simulink model "TwoLevelConverterIdealExample_HDL"  (R2023a)
settings: Solver=FixedStepAuto  StartTime=0.0  StopTime=0.1  RelTol=1e-3
PreLoadFcn:
  | ts = 1e-5; % local solver sample period
  | fsw = 1e3; % switching frequency
InitFcn:
  | load('stateSpaceParameters.mat');
undefined symbols (not defined in the file): DiscIntNeverNeededParam, ee_sli_rtmsupport, gcbh, stateSpaceParameters_1
libraries: fpga_utils_lib x5, hdlssclib x4, simulink x1, hdlsllib x1, eePwmGeneratorTwoLevel x1
settings Model: Creator=promero  LastModifiedBy=promero
settings OptimizationCC: BlockReduction=off  ConditionallyExecuteInputs=off  DefaultParameterBehavior=Inlined
settings DebuggingCC: AlgebraicLoopMsg=error
settings HardwareCC: ProdBitPerPointer=32  ProdBitPerSizeT=32  ProdBitPerPtrDiffT=32  ProdLargestAtomicFloat=None  ProdIntDivRoundTo=Undefined  ProdEndianess=Unspecified  ProdWordSize=32  ProdHWDeviceType=ASIC/FPGA->ASIC/FPGA  TargetBitPerPointer=64  TargetBitPerSizeT=64  TargetBitPerPtrDiffT=64  TargetLongLongMode=on  TargetIntDivRoundTo=Zero  TargetEndianess=LittleEndian  TargetWordSize=64  TargetHWDeviceType=Custom Processor->MATLAB Host Computer  ProdEqTarget=off

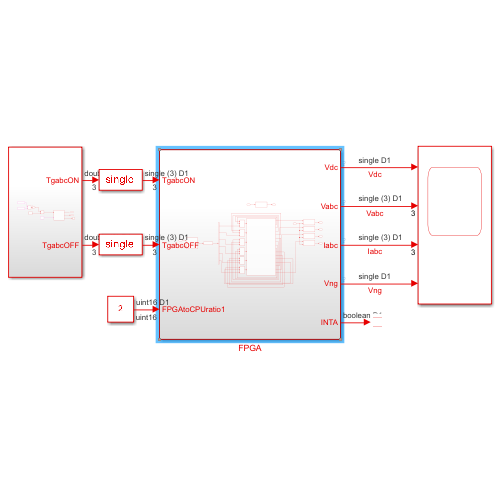
[thumbnail: Simulink's stored preview of the top-level diagram]
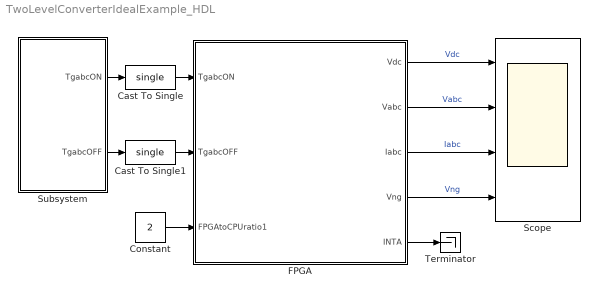
== system TwoLevelConverterIdealExample_HDL ==
  Cast To Single : DataTypeConversion  OutDataTypeStr=single  SaturateOnIntegerOverflow=off  RndMeth=Floor
  Cast To Single1 : DataTypeConversion  OutDataTypeStr=single  SaturateOnIntegerOverflow=off  RndMeth=Floor
  Constant : Constant  Value=2  OutDataTypeStr=uint16  SampleTime=-1
  FPGA : Subsystem
  Scope : Scope  NumInputPorts=4
  Subsystem : Subsystem
  Terminator : Terminator
  wires:
  FPGA/1(Vdc) -> Scope/1  "Vdc"
  FPGA/2(Vabc) -> Scope/2  "Vabc"
  FPGA/3(Iabc) -> Scope/3  "Iabc"
  FPGA/4(Vng) -> Scope/4  "Vng"
  Subsystem/1(TgabcON) -> Cast To Single/1
  Subsystem/2(TgabcOFF) -> Cast To Single1/1
  Cast To Single/1 -> FPGA/1(TgabcON)
  Cast To Single1/1 -> FPGA/2(TgabcOFF)
  FPGA/5(INTA) -> Terminator/1
  Constant/1 -> FPGA/3(FPGAtoCPUratio1)

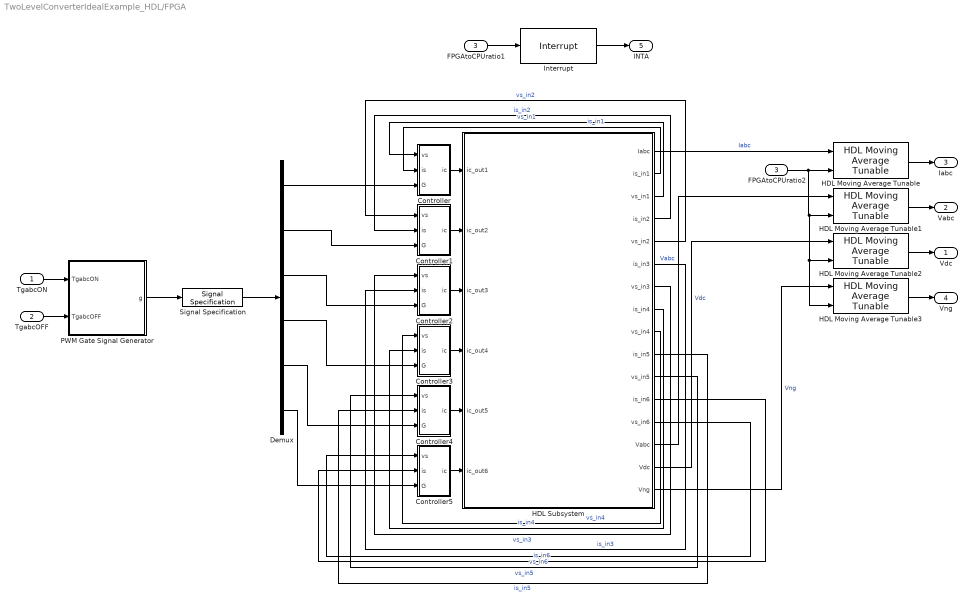
== system TwoLevelConverterIdealExample_HDL/FPGA ==
  TgabcON : Inport
  TgabcOFF : Inport  Port=2
  FPGAtoCPUratio1 : Inport  Port=3  OutDataTypeStr=uint16  LockScale=on
  Controller : Subsystem  mask{threshold=0.5, Gs=1e-6, s=1}
      mask prompts: Gs "Conductance (1/Ohm)"; s "Time scaling"
      mask DialogControl DescGroupVar Prompt: Description
      mask DialogControl Details Prompt: Switch Controller
  Controller1 : Subsystem  mask{threshold=0.5, Gs=1e-6, s=1}
      mask prompts: Gs "Conductance (1/Ohm)"; s "Time scaling"
      mask DialogControl DescGroupVar Prompt: Description
      mask DialogControl Details Prompt: Switch Controller
  Controller2 : Subsystem  mask{threshold=0.5, Gs=1e-6, s=1}
      mask prompts: Gs "Conductance (1/Ohm)"; s "Time scaling"
      mask DialogControl DescGroupVar Prompt: Description
      mask DialogControl Details Prompt: Switch Controller
  Controller3 : Subsystem  mask{threshold=0.5, Gs=1e-6, s=1}
      mask prompts: Gs "Conductance (1/Ohm)"; s "Time scaling"
      mask DialogControl DescGroupVar Prompt: Description
      mask DialogControl Details Prompt: Switch Controller
  Controller4 : Subsystem  mask{threshold=0.5, Gs=1e-6, s=1}
      mask prompts: Gs "Conductance (1/Ohm)"; s "Time scaling"
      mask DialogControl DescGroupVar Prompt: Description
      mask DialogControl Details Prompt: Switch Controller
  Controller5 : Subsystem  mask{threshold=0.5, Gs=1e-6, s=1}
      mask prompts: Gs "Conductance (1/Ohm)"; s "Time scaling"
      mask DialogControl DescGroupVar Prompt: Description
      mask DialogControl Details Prompt: Switch Controller
  Demux : Demux  Outputs=6
  FPGAtoCPUratio2 : InportShadow  Port=3  OutDataTypeStr=uint16
      settings: LockScale=on
  HDL Moving Average Tunable{,1..3} (4 alike) : fpga_utils_lib/HDL Moving Average Tunable  SystemSampleTime=-1  VariantActivationTime=update diagram  Latency=0  AutoFrameSizeCalculation=off
  HDL Subsystem : Subsystem  VariantControl=HDLSubsys
  Interrupt : fpga_utils_lib/Interrupt  SystemSampleTime=-1  VariantActivationTime=update diagram  Latency=0  AutoFrameSizeCalculation=off
  PWM Gate Signal Generator : Subsystem  Variant=on  VariantControlMode=label  VariantControl=Choice  LabelModeActiveChoice=hdlVar
  Signal Specification : SignalSpecification  OutDataTypeStr=boolean
      settings: LockScale=on
  Vdc : Outport
  Vabc : Outport  Port=2
  Iabc : Outport  Port=3
  Vng : Outport  Port=4
  INTA : Outport  Port=5
  wires:
  HDL Subsystem/3(vs_in1) -> Controller/1(vs)  "vs_in1"
  HDL Subsystem/7(vs_in3) -> Controller2/1(vs)  "vs_in3"
  Controller4/1(ic) -> HDL Subsystem/5(ic_out5)
  HDL Subsystem/5(vs_in2) -> Controller1/1(vs)  "vs_in2"
  Controller2/1(ic) -> HDL Subsystem/3(ic_out3)
  Controller/1(ic) -> HDL Subsystem/1(ic_out1)
  HDL Subsystem/2(is_in1) -> Controller/2(is)  "is_in1"
  HDL Subsystem/9(vs_in4) -> Controller3/1(vs)  "vs_in4"
  HDL Subsystem/12(is_in6) -> Controller5/2(is)  "is_in6"
  Controller5/1(ic) -> HDL Subsystem/6(ic_out6)
  Controller3/1(ic) -> HDL Subsystem/4(ic_out4)
  HDL Subsystem/4(is_in2) -> Controller1/2(is)  "is_in2"
  Controller1/1(ic) -> HDL Subsystem/2(ic_out2)
  Demux/1 -> Controller/3(G)
  HDL Subsystem/6(is_in3) -> Controller2/2(is)  "is_in3"
  HDL Subsystem/8(is_in4) -> Controller3/2(is)  "is_in4"
  HDL Subsystem/11(vs_in5) -> Controller4/1(vs)  "vs_in5"
  Demux/2 -> Controller1/3(G)
  HDL Subsystem/10(is_in5) -> Controller4/2(is)  "is_in5"
  Demux/3 -> Controller2/3(G)
  HDL Subsystem/13(vs_in6) -> Controller5/1(vs)  "vs_in6"
  Demux/6 -> Controller5/3(G)
  Demux/4 -> Controller3/3(G)
  Demux/5 -> Controller4/3(G)
  TgabcON/1 -> PWM Gate Signal Generator/1(TgabcON)
  TgabcOFF/1 -> PWM Gate Signal Generator/2(TgabcOFF)
  PWM Gate Signal Generator/1(g) -> Signal Specification/1
  Signal Specification/1 -> Demux/1
  Interrupt/1 -> INTA/1
  FPGAtoCPUratio1/1 -> Interrupt/1
  HDL Subsystem/1(Iabc) -> HDL Moving Average Tunable/1  "Iabc"
  FPGAtoCPUratio2/1 -> HDL Moving Average Tunable3/2, HDL Moving Average Tunable2/2, HDL Moving Average Tunable1/2, HDL Moving Average Tunable/2
  HDL Moving Average Tunable/1 -> Iabc/1
  HDL Subsystem/14(Vabc) -> HDL Moving Average Tunable1/1  "Vabc"
  HDL Subsystem/15(Vdc) -> HDL Moving Average Tunable2/1  "Vdc"
  HDL Subsystem/16(Vng) -> HDL Moving Average Tunable3/1  "Vng"
  HDL Moving Average Tunable1/1 -> Vabc/1
  HDL Moving Average Tunable2/1 -> Vdc/1
  HDL Moving Average Tunable3/1 -> Vng/1

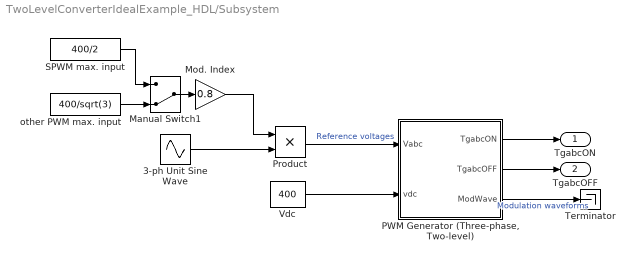
== system TwoLevelConverterIdealExample_HDL/Subsystem ==
  3-ph Unit Sine Wave : Sin  Frequency=2*pi*60  Phase="[0  -2*pi/3  2*pi/3] + pi/2"  SampleTime=ts
  Manual Switch1 : ManualSwitch  CurrentSetting=0
  Mod. Index : Gain  Gain=0.8
  "PWM Generator (Three-phase, Two-level)" : Subsystem  AncestorBlock=|  LoadFcn=ee_sli_rtmsupport( 'loadfcn', gcbh );  mask(PWM Generator (three-phase, two-level)){PWMMode=Continuous PWM (CPWM), CPWMMode=SVM: space vector modulation, DPWMMode=120 DPWM: positive dc component, SamplingMode=Natural, fsw=fsw, Ts=ts}
      | eePwmGeneratorTwoLevel/PWM Generator
      | (Three-phase, Two-level)
      mask prompts: PWMMode "physmod:ee:library:comments:control:eePwmGeneratorTwoLevel:PWMMode_MP"; CPWMMode "physmod:ee:library:comments:control:eePwmGeneratorTwoLevel:ContinuousPWM_MP"; DPWMMode "physmod:ee:library:comments:control:eePwmGeneratorTwoLevel:DiscontinuousPWM_MP"; SamplingMode "physmod:ee:library:comments:control:eePwmGeneratorTwoLevel:SamplingMode_MP"; fsw "physmod:ee:library:comments:control:eePwmGeneratorTwoLevel:SwitchingFrequencyHz_MP"; Ts "physmod:ee:library:comments:control:eePwmGeneratorTwoLevel:SampleTimes_MP"
      mask help: physmod:ee:library:comments:control:eePwmGeneratorTwoLevel:PWMGeneratorthreephaseTwolevel_MD
      mask init:
      | Tsw = 1/fsw;
      | 
      | if fsw <= 0
      |     error(message('physmod:simscape:compiler:patterns:checks:GreaterThanZero',getString(message('physmod:ee:library:comments:control:eePwmGeneratorTwoLevel:SwitchingFrequencyHz_MP'))));
      | end
      | 
      | if Ts <= 0
      |     error(message('physmod:simscape:compiler:patterns:checks:GreaterThanZero',getString(message('physmod:ee:library:comments:control:eePwmGeneratorTwoLevel:SampleTimes_MP'))));
      | end
      | 
      | if Ts > 1/(10*fsw)
      |     error(message('physmod:simscape:compiler:patterns:checks:LessThanOrEqual',getString(message('physmod:ee:library:comments:control:eePwmGeneratorTwoLevel:SampleTimes_MP')),getString(message('physmod:ee:library:comments:control:eePwmGeneratorTwoLevel:inverseOf10TimesSwitchingFrequency_MP'))));
      | end
      | 
      | switch SamplingMode
      |     case 'Natural'
      |         RateTransitionOnInput = -1;
      |         GateGeneratorX0 = 0;
      |     case 'Asymmetric'
      |         RateTransitionOnInput = 0.5*Tsw;
      |         GateGeneratorX0 = 0.5/fsw;
      |     case 'Symmetric'
      |         RateTransitionOnInput = Tsw;
      |         GateGeneratorX0 = 0;
      | end
      | 
      | 
      | switch PWMMode
      |     case 'Continuous PWM (CPWM)'
      |         switch CPWMMode
      |             case 'SPWM: sinusoidal PWM'
      |                 PWM = 1;
      |             case 'SVM: space vector modulation'
      |                 PWM = 2;
      |         end
      |     case 'Discontinuous PWM (DPWM)'
      |         switch DPWMMode
      |             case '60 DPWM: 60 degree discontinuous PWM'
      |                 PWM = 3;
      |             case '60 DPWM (+30 degree shift): +30 degree shift from 60 DPWM'
      |                 PWM = 4;
      |             case '60 DPWM (-30 degree shift): -30 degree shift from 60 DPWM'
      |                 PWM = 5;
      |             case '30 DPWM: 30 degree discontinuous PWM'
      |                 PWM = 6;
      |             case '120 DPWM: positive dc component'
      |                 PWM = 7;
      |             case '120 DPWM: negative dc component'
      |                 PWM = 8;
      |         end
      | end
      settings: CopyFcn=ee_sli_rtmsupport( 'copyfcn', gcbh );  DeleteFcn=ee_sli_rtmsupport( 'deletefcn', gcbh );  ModelCloseFcn=ee_sli_rtmsupport( 'modelclosefcn', gcbh );  PreSaveFcn=%pe_sli_rtmsupport( 'presavefcn', gcbh );  PostSaveFcn=ee_sli_rtmsupport( 'postsavefcn', gcbh );  PreCopyFcn=ee_sli_rtmsupport( 'precopyfcn', gcbh );  OpenFcn=ee_sli_rtmsupport( 'openfcn', gcbh );  CloseFcn=ee_sli_rtmsupport( 'closefcn', gcbh );  PreDeleteFcn=ee_sli_rtmsupport( 'predeletefcn', gcbh );
      settings: LibrarySourceBlock=|
      | eePwmGeneratorTwoLevel/PWM Generator
      | (Three-phase, Two-level)
      mask Help: web(nesl_help(gcbh))
      mask TypeOptions PWMMode: physmod:ee:library:comments:control:eePwmGeneratorTwoLevel:ContinuousPWMCPWM_PV | physmod:ee:library:comments:control:eePwmGeneratorTwoLevel:DiscontinuousPWMDPWM_PV
      mask Callback PWMMode:
      | switch get_param(gcb,'PWMMode')
      |     case 'Continuous PWM (CPWM)'
      |         set_param(gcb,'MaskVisibilities',{'on';'on';'off';'on';'on';'on'})
      |     case 'Discontinuous PWM (DPWM)'
      |         set_param(gcb,'MaskVisibilities',{'on';'off';'on';'on';'on';'on'})
      | end
      mask TypeOptions CPWMMode: physmod:ee:library:comments:control:eePwmGeneratorTwoLevel:SPWMSinusoidalPWM_PV | physmod:ee:library:comments:control:eePwmGeneratorTwoLevel:SVMSpaceVectorModulation_PV
      mask TypeOptions DPWMMode: physmod:ee:library:comments:control:eePwmGeneratorTwoLevel:x60DPWM60DegreeDiscontinuousPWM_PV | physmod:ee:library:comments:control:eePwmGeneratorTwoLevel:x60DPWM30DegreeShift30DegreeShiftFrom60DPWM_PV | physmod:ee:library:comments:control:eePwmGeneratorTwoLevel:x60DPWM0x2D30DegreeShift0x2D30DegreeShiftFrom60DPWM_PV | physmod:ee:library:comments:control:eePwmGeneratorTwoLevel:x30DPWM30DegreeDiscontinuousPWM_PV | physmod:ee:library:comments:control:eePwmGeneratorTwoLevel:x120DPWMPositiveDcComponent_PV | physmod:ee:library:comments:control:eePwmGeneratorTwoLevel:x120DPWMNegativeDcComponent_PV
      mask TypeOptions SamplingMode: physmod:ee:library:comments:control:eePwmGeneratorTwoLevel:Natural_PV | physmod:ee:library:comments:control:eePwmGeneratorTwoLevel:Asymmetric_PV | physmod:ee:library:comments:control:eePwmGeneratorTwoLevel:Symmetric_PV
      mask DialogControl ParameterGroupVar Prompt: physmod:ee:library:comments:control:eePwmGeneratorTwoLevel:tab_Parameters
      mask DialogControl PWMMode Prompt: PWM mode
      mask DialogControl CPWMMode Prompt: Continuous PWM
      mask DialogControl DPWMMode Prompt: Discontinuous PWM
      mask DialogControl SamplingMode Prompt: Sampling mode
      mask DialogControl fsw Prompt: Switching frequency (Hz)
      mask DialogControl Ts Prompt: Sample time (s)
  Product : Product
  SPWM max. input : Constant  Value=400/2
  Terminator : Terminator
  Vdc : Constant  Value=400
  other PWM max. input : Constant  Value=400/sqrt(3)
  TgabcON : Outport
  TgabcOFF : Outport  Port=2
  wires:
  Product/1 -> "PWM Generator (Three-phase, Two-level)"/1(Vabc)  "Reference voltages"
  Vdc/1 -> "PWM Generator (Three-phase, Two-level)"/2(vdc)
  other PWM max. input/1 -> Manual Switch1/2
  SPWM max. input/1 -> Manual Switch1/1
  Manual Switch1/1 -> Mod. Index/1
  "PWM Generator (Three-phase, Two-level)"/3(ModWave) -> Terminator/1  "Modulation waveforms"
  Mod. Index/1 -> Product/1
  3-ph Unit Sine Wave/1 -> Product/2
  "PWM Generator (Three-phase, Two-level)"/2(TgabcOFF) -> TgabcOFF/1
  "PWM Generator (Three-phase, Two-level)"/1(TgabcON) -> TgabcON/1

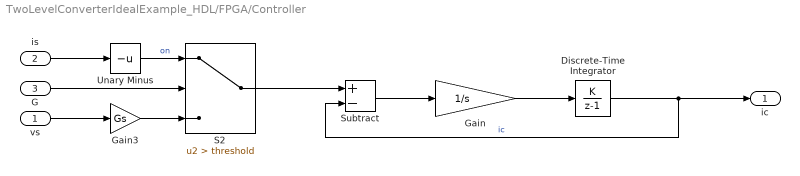
== system TwoLevelConverterIdealExample_HDL/FPGA/Controller ==
  vs : Inport
  is : Inport  Port=2
  G : Inport  Port=3
  Discrete-Time Integrator : DiscreteIntegrator  IntegratorMethod=Accumulation: Forward Euler  SampleTime=-1  ICPrevOutput=DiscIntNeverNeededParam  ICPrevScaledInput=DiscIntNeverNeededParam
  Gain : Gain  Gain=1/s
  Gain3 : Gain  Gain=Gs
  S2 : Switch  Criteria=u2 > Threshold  Threshold=threshold  SaturateOnIntegerOverflow=off  InputSameDT=off
  Subtract : Sum  Inputs=+-
  Unary Minus : UnaryMinus
  ic : Outport
  wires:
  G/1 -> S2/2
  is/1 -> Unary Minus/1
  Discrete-Time Integrator/1 -> Subtract/2, ic/1  "ic"
  Subtract/1 -> Gain/1
  Gain/1 -> Discrete-Time Integrator/1
  vs/1 -> Gain3/1
  S2/1 -> Subtract/1
  Gain3/1 -> S2/3
  Unary Minus/1 -> S2/1  "on"

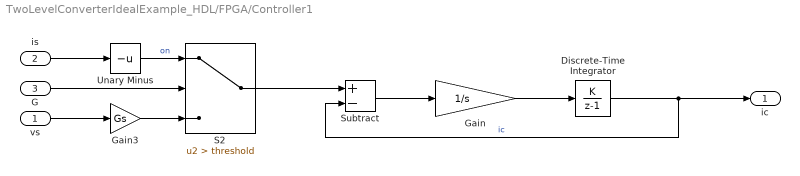
== system TwoLevelConverterIdealExample_HDL/FPGA/Controller1 ==
  vs : Inport
  is : Inport  Port=2
  G : Inport  Port=3
  Discrete-Time Integrator : DiscreteIntegrator  IntegratorMethod=Accumulation: Forward Euler  SampleTime=-1  ICPrevOutput=DiscIntNeverNeededParam  ICPrevScaledInput=DiscIntNeverNeededParam
  Gain : Gain  Gain=1/s
  Gain3 : Gain  Gain=Gs
  S2 : Switch  Criteria=u2 > Threshold  Threshold=threshold  SaturateOnIntegerOverflow=off  InputSameDT=off
  Subtract : Sum  Inputs=+-
  Unary Minus : UnaryMinus
  ic : Outport
  wires:
  Unary Minus/1 -> S2/1  "on"
  Gain3/1 -> S2/3
  S2/1 -> Subtract/1
  vs/1 -> Gain3/1
  Gain/1 -> Discrete-Time Integrator/1
  Subtract/1 -> Gain/1
  Discrete-Time Integrator/1 -> ic/1, Subtract/2  "ic"
  is/1 -> Unary Minus/1
  G/1 -> S2/2

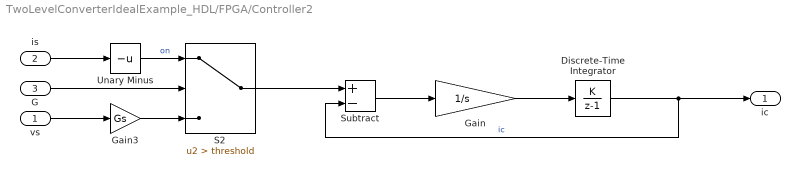
== system TwoLevelConverterIdealExample_HDL/FPGA/Controller2 ==
  vs : Inport
  is : Inport  Port=2
  G : Inport  Port=3
  Discrete-Time Integrator : DiscreteIntegrator  IntegratorMethod=Accumulation: Forward Euler  SampleTime=-1  ICPrevOutput=DiscIntNeverNeededParam  ICPrevScaledInput=DiscIntNeverNeededParam
  Gain : Gain  Gain=1/s
  Gain3 : Gain  Gain=Gs
  S2 : Switch  Criteria=u2 > Threshold  Threshold=threshold  SaturateOnIntegerOverflow=off  InputSameDT=off
  Subtract : Sum  Inputs=+-
  Unary Minus : UnaryMinus
  ic : Outport
  wires:
  Unary Minus/1 -> S2/1  "on"
  Gain3/1 -> S2/3
  S2/1 -> Subtract/1
  vs/1 -> Gain3/1
  Gain/1 -> Discrete-Time Integrator/1
  Subtract/1 -> Gain/1
  Discrete-Time Integrator/1 -> ic/1, Subtract/2  "ic"
  is/1 -> Unary Minus/1
  G/1 -> S2/2

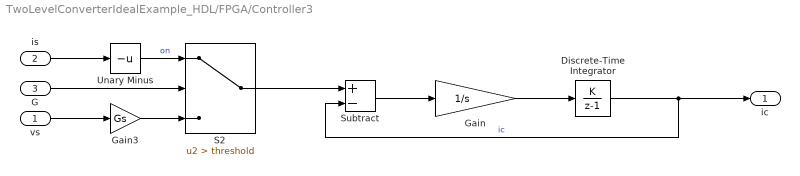
== system TwoLevelConverterIdealExample_HDL/FPGA/Controller3 ==
  vs : Inport
  is : Inport  Port=2
  G : Inport  Port=3
  Discrete-Time Integrator : DiscreteIntegrator  IntegratorMethod=Accumulation: Forward Euler  SampleTime=-1  ICPrevOutput=DiscIntNeverNeededParam  ICPrevScaledInput=DiscIntNeverNeededParam
  Gain : Gain  Gain=1/s
  Gain3 : Gain  Gain=Gs
  S2 : Switch  Criteria=u2 > Threshold  Threshold=threshold  SaturateOnIntegerOverflow=off  InputSameDT=off
  Subtract : Sum  Inputs=+-
  Unary Minus : UnaryMinus
  ic : Outport
  wires:
  G/1 -> S2/2
  is/1 -> Unary Minus/1
  Discrete-Time Integrator/1 -> Subtract/2, ic/1  "ic"
  Subtract/1 -> Gain/1
  Gain/1 -> Discrete-Time Integrator/1
  vs/1 -> Gain3/1
  S2/1 -> Subtract/1
  Gain3/1 -> S2/3
  Unary Minus/1 -> S2/1  "on"

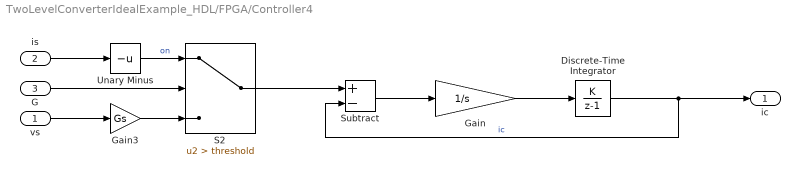
== system TwoLevelConverterIdealExample_HDL/FPGA/Controller4 ==
  vs : Inport
  is : Inport  Port=2
  G : Inport  Port=3
  Discrete-Time Integrator : DiscreteIntegrator  IntegratorMethod=Accumulation: Forward Euler  SampleTime=-1  ICPrevOutput=DiscIntNeverNeededParam  ICPrevScaledInput=DiscIntNeverNeededParam
  Gain : Gain  Gain=1/s
  Gain3 : Gain  Gain=Gs
  S2 : Switch  Criteria=u2 > Threshold  Threshold=threshold  SaturateOnIntegerOverflow=off  InputSameDT=off
  Subtract : Sum  Inputs=+-
  Unary Minus : UnaryMinus
  ic : Outport
  wires:
  G/1 -> S2/2
  is/1 -> Unary Minus/1
  Discrete-Time Integrator/1 -> Subtract/2, ic/1  "ic"
  Subtract/1 -> Gain/1
  Gain/1 -> Discrete-Time Integrator/1
  vs/1 -> Gain3/1
  S2/1 -> Subtract/1
  Gain3/1 -> S2/3
  Unary Minus/1 -> S2/1  "on"

== system TwoLevelConverterIdealExample_HDL/FPGA/Controller5 ==
  vs : Inport
  is : Inport  Port=2
  G : Inport  Port=3
  Discrete-Time Integrator : DiscreteIntegrator  IntegratorMethod=Accumulation: Forward Euler  SampleTime=-1  ICPrevOutput=DiscIntNeverNeededParam  ICPrevScaledInput=DiscIntNeverNeededParam
  Gain : Gain  Gain=1/s
  Gain3 : Gain  Gain=Gs
  S2 : Switch  Criteria=u2 > Threshold  Threshold=threshold  SaturateOnIntegerOverflow=off  InputSameDT=off
  Subtract : Sum  Inputs=+-
  Unary Minus : UnaryMinus
  ic : Outport
  wires:
  Unary Minus/1 -> S2/1  "on"
  Gain3/1 -> S2/3
  S2/1 -> Subtract/1
  vs/1 -> Gain3/1
  Gain/1 -> Discrete-Time Integrator/1
  Subtract/1 -> Gain/1
  Discrete-Time Integrator/1 -> ic/1, Subtract/2  "ic"
  is/1 -> Unary Minus/1
  G/1 -> S2/2

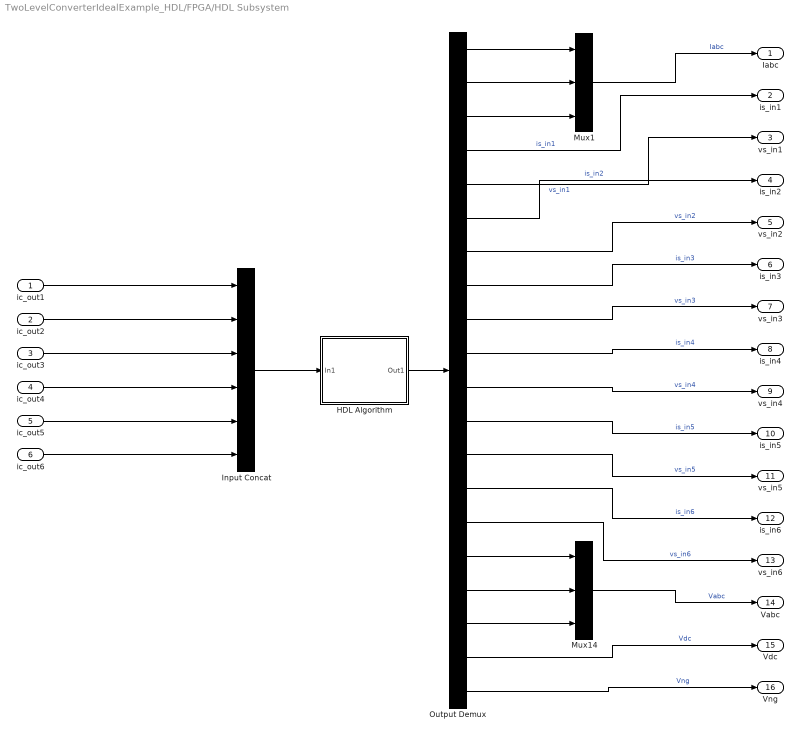
== system TwoLevelConverterIdealExample_HDL/FPGA/HDL Subsystem ==
  ic_out1 : Inport
  ic_out2 : Inport  Port=2
  ic_out3 : Inport  Port=3
  ic_out4 : Inport  Port=4
  ic_out5 : Inport  Port=5
  ic_out6 : Inport  Port=6
  HDL Algorithm : Subsystem  Variant=on  VariantControlMode=label  VariantControl=Choice  LabelModeActiveChoice=StateSpaceBlock
  Input Concat : Concatenate  NumInputs=6
  Mux1 : Mux  Inputs=3
  Mux14 : Mux  Inputs=3
  Output Demux : Demux  Outputs=20
  Iabc : Outport
  is_in1 : Outport  Port=2
  vs_in1 : Outport  Port=3
  is_in2 : Outport  Port=4
  vs_in2 : Outport  Port=5
  is_in3 : Outport  Port=6
  vs_in3 : Outport  Port=7
  is_in4 : Outport  Port=8
  vs_in4 : Outport  Port=9
  is_in5 : Outport  Port=10
  vs_in5 : Outport  Port=11
  is_in6 : Outport  Port=12
  vs_in6 : Outport  Port=13
  Vabc : Outport  Port=14
  Vdc : Outport  Port=15
  Vng : Outport  Port=16
  wires:
  Output Demux/7 -> vs_in2/1  "vs_in2"
  ic_out1/1 -> Input Concat/1
  Output Demux/18 -> Mux14/3
  Output Demux/17 -> Mux14/2
  Output Demux/16 -> Mux14/1
  Output Demux/13 -> vs_in5/1  "vs_in5"
  Output Demux/5 -> vs_in1/1  "vs_in1"
  Output Demux/2 -> Mux1/2
  Output Demux/19 -> Vdc/1  "Vdc"
  Output Demux/3 -> Mux1/3
  Output Demux/1 -> Mux1/1
  Output Demux/8 -> is_in3/1  "is_in3"
  Output Demux/10 -> is_in4/1  "is_in4"
  Mux1/1 -> Iabc/1  "Iabc"
  Output Demux/9 -> vs_in3/1  "vs_in3"
  Output Demux/15 -> vs_in6/1  "vs_in6"
  Output Demux/6 -> is_in2/1  "is_in2"
  Output Demux/4 -> is_in1/1  "is_in1"
  Output Demux/20 -> Vng/1  "Vng"
  ic_out3/1 -> Input Concat/3
  ic_out4/1 -> Input Concat/4
  ic_out5/1 -> Input Concat/5
  ic_out2/1 -> Input Concat/2
  Output Demux/11 -> vs_in4/1  "vs_in4"
  Output Demux/14 -> is_in6/1  "is_in6"
  Output Demux/12 -> is_in5/1  "is_in5"
  Mux14/1 -> Vabc/1  "Vabc"
  ic_out6/1 -> Input Concat/6
  Input Concat/1 -> HDL Algorithm/1(In1)
  HDL Algorithm/1(Out1) -> Output Demux/1

== system TwoLevelConverterIdealExample_HDL/FPGA/PWM Gate Signal Generator ==
  TgabcON : Inport
  TgabcOFF : Inport  Port=2
  HDL counter : Subsystem  VariantControl=hdlVar
      settings: LibrarySourceBlock=|
      | ee_sl_lib/Pulse Width
      | Modulation/PWM Gate Signal Generator
      | (Three-phase, Two-level)
  Off-the-shelf block : eePwmGeneratorTwoLevel/PWM Gate Signal Generator (Three-phase, Two-level)  VariantControl=defVar  fsw=fsw  Ts=ts
      settings: SamplingMode=Natural
      settings: LibrarySourceBlock=|
      | ee_sl_lib/Pulse Width
      | Modulation/PWM Gate Signal Generator
      | (Three-phase, Two-level)
  g : Outport

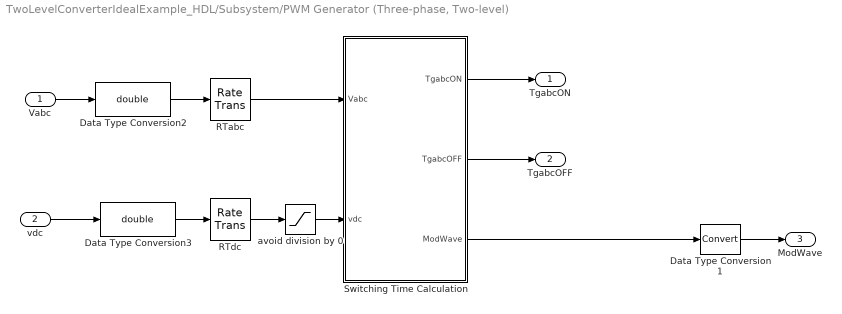
== system TwoLevelConverterIdealExample_HDL/Subsystem/PWM Generator (Three-phase, Two-level) ==
  Vabc : Inport
  vdc : Inport  Port=2
  Data Type Conversion1 : DataTypeConversion  SaturateOnIntegerOverflow=off  RndMeth=Floor
  Data Type Conversion2 : DataTypeConversion  OutDataTypeStr=double  SaturateOnIntegerOverflow=off  RndMeth=Floor
  Data Type Conversion3 : DataTypeConversion  OutDataTypeStr=double  SaturateOnIntegerOverflow=off  RndMeth=Floor
  RTabc : RateTransition  OutPortSampleTime=RateTransitionOnInput
  RTdc : RateTransition  OutPortSampleTime=RateTransitionOnInput
  Switching Time Calculation : MATLAB Function  TreatAsAtomicUnit=on
  avoid division by 0 : Saturate  UpperLimit=inf  LowerLimit=eps
  TgabcON : Outport
  TgabcOFF : Outport  Port=2
  ModWave : Outport  Port=3  VectorParamsAs1DForOutWhenUnconnected=off
  wires:
  Data Type Conversion3/1 -> RTdc/1
  Data Type Conversion2/1 -> RTabc/1
  vdc/1 -> Data Type Conversion3/1
  Vabc/1 -> Data Type Conversion2/1
  Switching Time Calculation/1(TgabcON) -> TgabcON/1
  Switching Time Calculation/2(TgabcOFF) -> TgabcOFF/1
  Switching Time Calculation/3(ModWave) -> Data Type Conversion1/1
  RTabc/1 -> Switching Time Calculation/1(Vabc)
  RTdc/1 -> avoid division by 0/1
  avoid division by 0/1 -> Switching Time Calculation/2(vdc)
  Data Type Conversion1/1 -> ModWave/1

== system TwoLevelConverterIdealExample_HDL/FPGA/HDL Subsystem/HDL Algorithm ==
  In1 : Inport
  HDL Algorithm : Subsystem  VariantControl=HDL
  State-Space Block : Subsystem  VariantControl=StateSpaceBlock
  Out1 : Outport

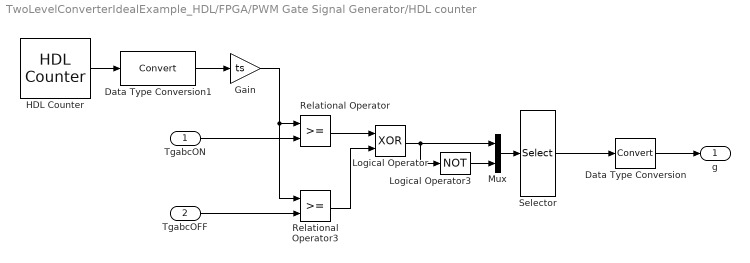
== system TwoLevelConverterIdealExample_HDL/FPGA/PWM Gate Signal Generator/HDL counter ==
  TgabcON : Inport
  TgabcOFF : Inport  Port=2
  Data Type Conversion : DataTypeConversion  SaturateOnIntegerOverflow=off  RndMeth=Floor
  Data Type Conversion1 : DataTypeConversion  SaturateOnIntegerOverflow=off  RndMeth=Floor
  Gain : Gain  Gain=ts
  HDL Counter : hdlsllib/Sources/HDL Counter  CountType=Count limited  CountInit=0  CountStep=1  CountMax=floor(1/fsw/ts-1)  CountFromType=Initial value  CountFrom=0  CountResetPort=off  CountLoadPort=off  CountEnbPort=off  CountDirPort=off  CountHitOutputPort=off  CountDataType=Unsigned  CountWordLen=16  CountFracLen=0  CountSampTime=ts
  Logical Operator : Logic  Operator=XOR  AllPortsSameDT=off  OutDataTypeStr=boolean
  Logical Operator3 : Logic  Operator=NOT  AllPortsSameDT=off  OutDataTypeStr=boolean
  Mux : Mux  Inputs=2
  Relational Operator : RelationalOperator  OutDataTypeStr=boolean
  Relational Operator3 : RelationalOperator  OutDataTypeStr=boolean
  Selector : Selector  InputPortWidth=6  IndexOptions=Index vector (dialog)  Indices=[1 4 2 5 3 6]  OutputSizes=1
  g : Outport  VectorParamsAs1DForOutWhenUnconnected=off
  wires:
  Data Type Conversion/1 -> g/1
  Relational Operator/1 -> Logical Operator/1
  Logical Operator3/1 -> Mux/2
  Relational Operator3/1 -> Logical Operator/2
  TgabcOFF/1 -> Relational Operator3/2
  Logical Operator/1 -> Mux/1, Logical Operator3/1
  Selector/1 -> Data Type Conversion/1
  Gain/1 -> Relational Operator/1, Relational Operator3/1
  Mux/1 -> Selector/1
  TgabcON/1 -> Relational Operator/2
  HDL Counter/1 -> Data Type Conversion1/1
  Data Type Conversion1/1 -> Gain/1

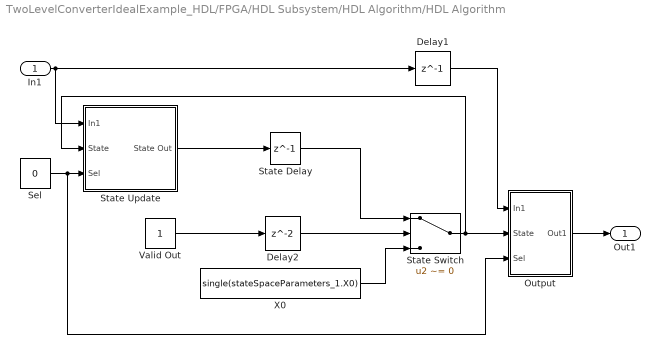
== system TwoLevelConverterIdealExample_HDL/FPGA/HDL Subsystem/HDL Algorithm/HDL Algorithm ==
  In1 : Inport
  Delay1 : Delay  DelayLength=1
  Delay2 : Delay
  Output : Subsystem
  Sel : Constant  Value=0  OutDataTypeStr=uint32  SampleTime=-1
  State Delay : Delay  DelayLength=1  InitialCondition=single(stateSpaceParameters_1.X0)
  State Switch : Switch  Criteria=u2 ~= 0  SaturateOnIntegerOverflow=off  InputSameDT=off
  State Update : Subsystem
  Valid Out : Constant  OutDataTypeStr=boolean  SampleTime=-1
  X0 : Constant  Value=single(stateSpaceParameters_1.X0)  SampleTime=-1
  Out1 : Outport  VectorParamsAs1DForOutWhenUnconnected=off
  wires:
  State Delay/1 -> State Switch/1
  In1/1 -> State Update/1(In1), Delay1/1
  X0/1 -> State Switch/3
  Sel/1 -> Output/3(Sel), State Update/3(Sel)
  Delay2/1 -> State Switch/2
  State Update/1(State Out) -> State Delay/1
  Valid Out/1 -> Delay2/1
  Delay1/1 -> Output/1(In1)
  State Switch/1 -> State Update/2(State), Output/2(State)
  Output/1(Out1) -> Out1/1

== system TwoLevelConverterIdealExample_HDL/FPGA/HDL Subsystem/HDL Algorithm/State-Space Block ==
  In1 : Inport
  Bias : Bias  Bias=stateSpaceParameters_1.Y0d  SaturateOnIntegerOverflow=off
  Fixed-Point State-Space : simulink/Additional Math & Discrete/Additional Discrete/Fixed-Point State-Space  A=stateSpaceParameters_1.Ad  B=stateSpaceParameters_1.Bd  C=stateSpaceParameters_1.Cd  D=stateSpaceParameters_1.Dd  InitialCondition=stateSpaceParameters_1.X0  InternalDataType=fixdt('single')  StateEqScaling=2^0  OutputEqScaling=2^0  DoSatur=off
  Signal Specification : SignalSpecification  OutDataTypeStr=single
  Out1 : Outport
  wires:
  In1/1 -> Signal Specification/1
  Fixed-Point State-Space/1 -> Bias/1
  Bias/1 -> Out1/1
  Signal Specification/1 -> Fixed-Point State-Space/1

== system TwoLevelConverterIdealExample_HDL/FPGA/HDL Subsystem/HDL Algorithm/HDL Algorithm/Output ==
  In1 : Inport
  State : Inport  Port=2
  Sel : Inport  Port=3
  Bias : Subsystem
  Multiply Input : hdlssclib/NFPSparseConstMultiply  constMatrix=single(stateSpaceParameters_1.Dd)
  Multiply State : hdlssclib/NFPSparseConstMultiply  constMatrix=single(stateSpaceParameters_1.Cd)
  Output Sum : Sum  Inputs=+++
  Out1 : Outport  VectorParamsAs1DForOutWhenUnconnected=off
  wires:
  State/1 -> Multiply State/1
  In1/1 -> Multiply Input/1
  Sel/1 -> Multiply State/2, Multiply Input/2, Bias/1(Sel)
  Output Sum/1 -> Out1/1
  Multiply Input/1 -> Output Sum/1
  Multiply State/1 -> Output Sum/2
  Bias/1(Out1) -> Output Sum/3

== system TwoLevelConverterIdealExample_HDL/FPGA/HDL Subsystem/HDL Algorithm/HDL Algorithm/State Update ==
  In1 : Inport
  State : Inport  Port=2
  Sel : Inport  Port=3
  Bias : Subsystem
  Multiply Input : hdlssclib/NFPSparseConstMultiply  constMatrix=single(stateSpaceParameters_1.Bd)
  Multiply State : hdlssclib/NFPSparseConstMultiply  constMatrix=single(stateSpaceParameters_1.Ad)
  Output Sum : Sum  Inputs=+++
  State Out : Outport  OutDataTypeStr=single  VectorParamsAs1DForOutWhenUnconnected=off
  wires:
  State/1 -> Multiply State/1
  In1/1 -> Multiply Input/1
  Sel/1 -> Multiply State/2, Multiply Input/2, Bias/1(Sel)
  Output Sum/1 -> State Out/1
  Multiply Input/1 -> Output Sum/1
  Multiply State/1 -> Output Sum/2
  Bias/1(Out1) -> Output Sum/3

== system TwoLevelConverterIdealExample_HDL/FPGA/HDL Subsystem/HDL Algorithm/HDL Algorithm/Output/Bias ==
  Sel : Inport
  Bias : Constant  Value=single(stateSpaceParameters_1.Y0d)  SampleTime=-1
  Terminator : Terminator
  Out1 : Outport  VectorParamsAs1DForOutWhenUnconnected=off
  wires:
  Sel/1 -> Terminator/1
  Bias/1 -> Out1/1

== system TwoLevelConverterIdealExample_HDL/FPGA/HDL Subsystem/HDL Algorithm/HDL Algorithm/State Update/Bias ==
  Sel : Inport
  Bias : Constant  Value=single(stateSpaceParameters_1.F0d)  SampleTime=-1
  Terminator : Terminator
  Out1 : Outport  VectorParamsAs1DForOutWhenUnconnected=off
  wires:
  Sel/1 -> Terminator/1
  Bias/1 -> Out1/1

== matlab function TwoLevelConverterIdealExample_HDL/Subsystem/PWM Generator (Three-phase, Two-level)/Switching Time Calculation ==
  settings: sampleTime=1
  data: Vabc input; TgabcON output; vdc input; TgabcOFF output; ModWave output; fsw parameter; PWM parameter
function [TgabcON,TgabcOFF,ModWave]  = switchingTime(Vabc,vdc,fsw,PWM)

[TgabcON,TgabcOFF,ModWave] = ee.control.pwmSwitchingTimeTwoLevel(Vabc,vdc,fsw,PWM);
